simulink model "model_base_bros"  (R2017b)
settings: Solver=FixedStepDiscrete  StartTime=0.0  StopTime=inf  FixedStep=sampleTime  RelTol=1e-3
PostLoadFcn:
  | % load model parameters
  | % pname = fileparts(get_param('model_base_bros','filename'));
  | % run([pname  '\parameters_base_model_bros.m']);
  | parameters_base_model_bros;
  | 
  | % set requested state
  | set_param('model_base_bros/Requested state','Value',num2str(0));
InitFcn:
  | % load model parameters
  | % pname = fileparts(get_param('model_base_bros','filename'));
  | % run([pname  '\parameters_base_model_bros.m']);
  | parameters_base_model_bros;
  | 
  | % set requested state
  | set_param('model_base_bros/Requested state','Value',num2str(0));
StartFcn:
  | % load model parameters
  | % pname = fileparts(get_param('model_base_bros','filename'));
  | % run([pname  '\parameters_base_model_bros.m']);
  | parameters_base_model_bros;
  | 
  | % set requested state
  | set_param('model_base_bros/Requested state','Value',num2str(0));
StopFcn:
  | % switch off data logger (to hopefully avoid corrupt files). TwinCAT doesn't properly switch off the logger when shutting down the model
  | % no idea if this'll work.
  | set_param('model_base_bros/Record data (1 = yes, 0 = no)','Value',num2str(0));
values from neighbouring files (symbols this model uses):
  FFMatrix = -[0 -15; 15 0]    [parameters_base_model_bros.m]
  Lb = 0.07    [parameters_base_model_bros.m]
  Lf = 0.238    [parameters_base_model_bros.m]
  Lu = 0.153    [parameters_base_model_bros.m]
  msin_data_dist1 = [5 11 19 41 59 71 101 137 179 227 0.0358569687947 0.0275584886584 ... (30 elements, 10x3)]    [forcingfunction_data_id.mat]    (also in forcingfunction_data_id_2d_var6_1.mat = [0 0 0 0 0 0 0 0 0 0 0 0 ... (60 elements, 10x6)]; forcingfunction_data_id_2d_var75_nt11.mat = [0 0 0 0 0 0 0 0 0 0 0 0 ... (60 elements, 10x6)]; forcingfunction_data_id_nt10_var6.mat = [5 11 19 41 59 71 101 137 179 227 0.0248424367031 0.01909308)
  msin_data_dist2 = [7 13 23 43 61 73 103 139 181 229 0.0366642780879 0.0272817537998 ... (30 elements, 10x3)]    [forcingfunction_data_id.mat]    (also in forcingfunction_data_id_2d_var6_1.mat = [0 0 0 0 0 0 0 0 0 0 0 0 ... (60 elements, 10x6)]; forcingfunction_data_id_2d_var75_nt11.mat = [0 0 0 0 0 0 0 0 0 0 0 0 ... (60 elements, 10x6)]; forcingfunction_data_id_nt10_var6.mat = [7 13 23 43 61 73 103 139 181 229 0.0254017569884 0.01890135)
  msin_data_target = [2 9 17 27 37 47 0.0347382902327 0.0275101923829 0.0180185190239 0.0110214159229 0.0075682474126 0.00574660779142 ... (18 elements, 6x3)]    [forcingfunction_data_id.mat]    (also in forcingfunction_data_id_2d_var6_1.mat = [5 11 23 37 51 71 101 137 171 226 0.0252651788023 0.01941798; forcingfunction_data_id_2d_var75_nt11.mat = [5 11 23 37 51 71 101 137 173 227 263 0.0282088788597 ... (6; forcingfunction_data_id_nt10_var6.mat = [2 9 17 29 37 47 67 107 149 211 0.0239780224904 0.0189888450; forcingfunction_id_emg.mat = [3 7 13 19 31 0.0450441024419 0.0275859409824 0.015205627144)
  sampleTime = 0.001    [parameters_base_model_bros.m]
  Tm = 81.92    [forcingfunction_data_id_2d_var6_1.mat]    (also in forcingfunction_data_id_2d_var75_nt11.mat; forcingfunction_data_id_nt10_var6.mat; forcingfunction_id_emg.mat = 24)
undefined symbols (not defined in the file or in its folder): BROS1, BROS2, DiscIntNeverNeededParam
libraries: simulink x28, LibraryFM x14, VariousBlocksLibrary x13, simulink_extras x1
(part 3 of 4)

== system model_base_bros/Robot2/DataToEtherCAT/WorkspacePositionGuard ==
  note: Check internal angles
  note: Check whether endpoint position is within the predefined workspace
      | (ellipse)
  note: Check for singularity of joint configuration by checking
      | the condition number. When it exceeds a certain value, go to a safe mode
      | For now, this means disabling the actuators.
      | Note that the boundaries set using admittance should prohibit this from happening.
      | However, if sometjhing really goes wrong, this is a safe guard
  BusRobot : Inport
  StateSystem : Inport  Port=2
  AvoidAlgebraicLoop : Memory
  Bus Selector : BusSelector  OutputSignals=xOpSpace.x,xOpSpace.conditioning,qJointSpace.q_all
  CheckInternalAngles : MATLAB Function  TreatAsAtomicUnit=on
  Compare To Constant : simulink/Logic and Bit Operations/Compare To Constant  relop=>  const=4  OutDataTypeStr=boolean
  Compare To Constant1 : simulink/Logic and Bit Operations/Compare To Constant  relop=>=  const=2.75  OutDataTypeStr=boolean
  Data Type Conversion1 : DataTypeConversion  OutDataTypeStr=boolean
  Data Type Conversion2 : DataTypeConversion  Commented=through  OutDataTypeStr=int32
  Data Type Conversion4 : DataTypeConversion  OutDataTypeStr=boolean
  Detect Change : simulink/Logic and Bit Operations/Detect Change  vinit=0  InputProcessing=Inherited  OutDataTypeStr=boolean
  EndpointPositionGuard : MATLAB Function  TreatAsAtomicUnit=on
  LatchRising : LibraryFM/Utilities/LatchRising  ic=0
  Logical Operator : Logic  Operator=OR  AllPortsSameDT=off  OutDataTypeStr=boolean
  Mux : Mux  Inputs=2
  ShowWorkspaceErrorLatched : Display
  WorkspaceLastError : Display
  WorkspaceError : Outport
  WorkspaceErrorLatched : Outport  Port=2
  wires:
  BusRobot/1 -> Bus Selector/1
  Bus Selector/1 -> EndpointPositionGuard/2(xe)  "<x>"
  LatchRising/1 -> Data Type Conversion2/1
  EndpointPositionGuard/1(error) -> Data Type Conversion1/1
  Mux/1 -> AvoidAlgebraicLoop/1, WorkspaceLastError/1
  Detect Change/1 -> LatchRising/Trigger
  AvoidAlgebraicLoop/1 -> WorkspaceError/1, Detect Change/1, LatchRising/1
  Compare To Constant/1 -> EndpointPositionGuard/1(correctState)
  Bus Selector/2 -> Compare To Constant1/1  "<conditioning>"
  StateSystem/1 -> Compare To Constant/1
  Data Type Conversion2/1 -> WorkspaceErrorLatched/1, ShowWorkspaceErrorLatched/1
  CheckInternalAngles/1(angleError) -> Data Type Conversion4/1
  Bus Selector/3 -> CheckInternalAngles/1(theta)  "<q_all>"
  Data Type Conversion4/1 -> Mux/2
  Logical Operator/1 -> Mux/1
  Data Type Conversion1/1 -> Logical Operator/1
  Compare To Constant1/1 -> Logical Operator/2

== system model_base_bros/Experiment & Haptics/Admittance // Virtual model1/Virtual Model/HoldFirstSampleOnEnable ==
  note: These blocks hold the first sample of the input
      | when the block is enabled (through the action port)
  x : Inport
  Enable : EnablePort  StatesWhenEnabling=reset
  Counter Free-Running : simulink/Sources/Counter Free-Running  NumBits=32  tsamp=-1
  Display : Display
  Memory1 : Memory
  Switch : Switch  Threshold=1
  x0 : Outport
  wires:
  Switch/1 -> Display/1, Memory1/1, x0/1
  Memory1/1 -> Switch/1
  Counter Free-Running/1 -> Switch/2
  x/1 -> Switch/3

== system model_base_bros/Experiment & Haptics/Admittance // Virtual model1/Virtual Model/HoldFirstSampleOnEnable1 ==
  note: These blocks hold the first sample of the input
      | when the block is enabled (through the action port)
  x : Inport
  Enable : EnablePort  StatesWhenEnabling=reset
  Counter Free-Running : simulink/Sources/Counter Free-Running  NumBits=32  tsamp=-1
  Display : Display
  Memory1 : Memory
  Switch : Switch  Threshold=1
  x0 : Outport
  wires:
  Switch/1 -> Display/1, Memory1/1, x0/1
  Memory1/1 -> Switch/1
  Counter Free-Running/1 -> Switch/2
  x/1 -> Switch/3

== system model_base_bros/Robot1/Controller_PD/at home/HoldFirstSampleOnEnable ==
  note: These blocks hold the first sample of the input
      | when the block is enabled (through the action port)
  x : Inport
  Enable : EnablePort  StatesWhenEnabling=reset
  Counter Free-Running : simulink/Sources/Counter Free-Running  NumBits=32  tsamp=-1
  Memory1 : Memory
  Signal Conversion : SignalConversion  OverrideOpt=off
  Switch : Switch  Threshold=1
  x0 : Outport
  wires:
  x/1 -> Switch/3
  Counter Free-Running/1 -> Switch/2
  Memory1/1 -> Switch/1
  Switch/1 -> Signal Conversion/1, Memory1/1
  Signal Conversion/1 -> x0/1

== system model_base_bros/Robot1/DataFromEtherCAT/Calculate Arrange Joint and Op Space/forward kinematics ==
  JointPosition_rad : Inport  PortDimensions=[2 1]
  JointVelocity_rads : Inport  Port=2  PortDimensions=[2 1]
  JointAcceleration_rads2 : Inport  Port=3  PortDimensions=[2 1]
  Je : MATLAB Function  TreatAsAtomicUnit=on
  Jedot : MATLAB Function  TreatAsAtomicUnit=on
  Product : Product  Multiplication=Matrix(*)
  calculate xddot : MATLAB Function  TreatAsAtomicUnit=on
  forward kinematics : MATLAB Function  TreatAsAtomicUnit=on
  x : Outport
  xdot : Outport  Port=2
  xddot : Outport  Port=3
  J : Outport  Port=4
  Jdot : Outport  Port=5
  wires:
  JointPosition_rad/1 -> forward kinematics/1(q), Jedot/1(q), Je/1(q)
  Je/1(Je) -> calculate xddot/3(J), Product/1, J/1
  JointVelocity_rads/1 -> calculate xddot/2(qdot), Product/2, Jedot/2(qdot)
  Jedot/1(Jedot) -> calculate xddot/4(Jdot), Jdot/1
  Product/1 -> xdot/1
  forward kinematics/1(x) -> x/1
  calculate xddot/1(xddot) -> xddot/1
  JointAcceleration_rads2/1 -> calculate xddot/1(qddot)

== system model_base_bros/Robot1/DataFromEtherCAT/Calculate Arrange Joint and Op Space/forward kinematics1 ==
  JointPosition_rad : Inport  PortDimensions=[2 1]
  JointVelocity_rads : Inport  Port=2  PortDimensions=[2 1]
  JointAcceleration_rads2 : Inport  Port=3  PortDimensions=[2 1]
  Je : MATLAB Function  TreatAsAtomicUnit=on
  Jedot : MATLAB Function  TreatAsAtomicUnit=on
  Product : Product  Multiplication=Matrix(*)
  calculate xddot : MATLAB Function  TreatAsAtomicUnit=on
  forward kinematics : MATLAB Function  TreatAsAtomicUnit=on
  x : Outport
  xdot : Outport  Port=2
  xddot : Outport  Port=3
  J : Outport  Port=4
  Jdot : Outport  Port=5
  wires:
  JointPosition_rad/1 -> forward kinematics/1(q), Jedot/1(q), Je/1(q)
  Je/1(Je) -> calculate xddot/3(J), Product/1, J/1
  JointVelocity_rads/1 -> calculate xddot/2(qdot), Product/2, Jedot/2(qdot)
  Jedot/1(Jedot) -> calculate xddot/4(Jdot), Jdot/1
  Product/1 -> xdot/1
  forward kinematics/1(x) -> x/1
  calculate xddot/1(xddot) -> xddot/1
  JointAcceleration_rads2/1 -> calculate xddot/1(qddot)

== system model_base_bros/Robot1/DataFromEtherCAT/FTSensor_K6D27/spikefilter ==
  in : Inport
  Demux : Demux  Outputs=6
  Mux1 : Mux  Inputs=6
  spike filter oeps : Subsystem
  spike filter oeps1 : Subsystem
  spike filter oeps2 : Subsystem
  spike filter oeps3 : Subsystem
  spike filter oeps4 : Subsystem
  spike filter oeps5 : Subsystem
  out : Outport
  wires:
  spike filter oeps1/1(y) -> Mux1/2
  Mux1/1 -> out/1
  in/1 -> Demux/1
  Demux/3 -> spike filter oeps2/1(u)
  spike filter oeps4/1(y) -> Mux1/5
  spike filter oeps/1(y) -> Mux1/1
  Demux/6 -> spike filter oeps5/1(u)
  spike filter oeps5/1(y) -> Mux1/6
  Demux/1 -> spike filter oeps/1(u)
  Demux/2 -> spike filter oeps1/1(u)
  Demux/4 -> spike filter oeps3/1(u)
  Demux/5 -> spike filter oeps4/1(u)
  spike filter oeps2/1(y) -> Mux1/3
  spike filter oeps3/1(y) -> Mux1/4

== system model_base_bros/Robot2/Controller_PD/at home/HoldFirstSampleOnEnable ==
  note: These blocks hold the first sample of the input
      | when the block is enabled (through the action port)
  x : Inport
  Enable : EnablePort  StatesWhenEnabling=reset
  Counter Free-Running : simulink/Sources/Counter Free-Running  NumBits=32  tsamp=-1
  Memory1 : Memory
  Signal Conversion : SignalConversion  OverrideOpt=off
  Switch : Switch  Threshold=1
  x0 : Outport
  wires:
  x/1 -> Switch/3
  Counter Free-Running/1 -> Switch/2
  Memory1/1 -> Switch/1
  Switch/1 -> Signal Conversion/1, Memory1/1
  Signal Conversion/1 -> x0/1

== system model_base_bros/Robot2/DataFromEtherCAT/Calculate Arrange Joint and Op Space/forward kinematics ==
  JointPosition_rad : Inport  PortDimensions=[2 1]
  JointVelocity_rads : Inport  Port=2  PortDimensions=[2 1]
  JointAcceleration_rads2 : Inport  Port=3  PortDimensions=[2 1]
  Je : MATLAB Function  TreatAsAtomicUnit=on
  Jedot : MATLAB Function  TreatAsAtomicUnit=on
  Product : Product  Multiplication=Matrix(*)
  calculate xddot : MATLAB Function  TreatAsAtomicUnit=on
  forward kinematics : MATLAB Function  TreatAsAtomicUnit=on
  x : Outport
  xdot : Outport  Port=2
  xddot : Outport  Port=3
  J : Outport  Port=4
  Jdot : Outport  Port=5
  wires:
  JointPosition_rad/1 -> forward kinematics/1(q), Jedot/1(q), Je/1(q)
  Je/1(Je) -> calculate xddot/3(J), Product/1, J/1
  JointVelocity_rads/1 -> calculate xddot/2(qdot), Product/2, Jedot/2(qdot)
  Jedot/1(Jedot) -> calculate xddot/4(Jdot), Jdot/1
  Product/1 -> xdot/1
  forward kinematics/1(x) -> x/1
  calculate xddot/1(xddot) -> xddot/1
  JointAcceleration_rads2/1 -> calculate xddot/1(qddot)

== system model_base_bros/Robot2/DataFromEtherCAT/Calculate Arrange Joint and Op Space/forward kinematics1 ==
  JointPosition_rad : Inport  PortDimensions=[2 1]
  JointVelocity_rads : Inport  Port=2  PortDimensions=[2 1]
  JointAcceleration_rads2 : Inport  Port=3  PortDimensions=[2 1]
  Je : MATLAB Function  TreatAsAtomicUnit=on
  Jedot : MATLAB Function  TreatAsAtomicUnit=on
  Product : Product  Multiplication=Matrix(*)
  calculate xddot : MATLAB Function  TreatAsAtomicUnit=on
  forward kinematics : MATLAB Function  TreatAsAtomicUnit=on
  x : Outport
  xdot : Outport  Port=2
  xddot : Outport  Port=3
  J : Outport  Port=4
  Jdot : Outport  Port=5
  wires:
  JointPosition_rad/1 -> forward kinematics/1(q), Jedot/1(q), Je/1(q)
  Je/1(Je) -> calculate xddot/3(J), Product/1, J/1
  JointVelocity_rads/1 -> calculate xddot/2(qdot), Product/2, Jedot/2(qdot)
  Jedot/1(Jedot) -> calculate xddot/4(Jdot), Jdot/1
  Product/1 -> xdot/1
  forward kinematics/1(x) -> x/1
  calculate xddot/1(xddot) -> xddot/1
  JointAcceleration_rads2/1 -> calculate xddot/1(qddot)

== system model_base_bros/Robot2/DataFromEtherCAT/FTSensor_K6D27/spikefilter ==
  in : Inport
  Demux : Demux  Outputs=6
  Mux1 : Mux  Inputs=6
  spike filter oeps : Subsystem
  spike filter oeps1 : Subsystem
  spike filter oeps2 : Subsystem
  spike filter oeps3 : Subsystem
  spike filter oeps4 : Subsystem
  spike filter oeps5 : Subsystem
  out : Outport
  wires:
  spike filter oeps1/1(y) -> Mux1/2
  Mux1/1 -> out/1
  in/1 -> Demux/1
  Demux/3 -> spike filter oeps2/1(u)
  spike filter oeps4/1(y) -> Mux1/5
  spike filter oeps/1(y) -> Mux1/1
  Demux/6 -> spike filter oeps5/1(u)
  spike filter oeps5/1(y) -> Mux1/6
  Demux/1 -> spike filter oeps/1(u)
  Demux/2 -> spike filter oeps1/1(u)
  Demux/4 -> spike filter oeps3/1(u)
  Demux/5 -> spike filter oeps4/1(u)
  spike filter oeps2/1(y) -> Mux1/3
  spike filter oeps3/1(y) -> Mux1/4

== system model_base_bros/Robot1/DataFromEtherCAT/FTSensor_K6D27/spikefilter/spike filter oeps ==
  u : Inport
  'oeps' filter : MATLAB Function  TreatAsAtomicUnit=on
  Memory : Memory
  Terminator : Terminator
  diff threshold spike : Constant  Value=FTSensorStruct.ThresholdDiffForceSensorSpike
  y : Outport
  wires:
  'oeps' filter/2(y) -> y/1, Memory/1
  diff threshold spike/1 -> 'oeps' filter/2(diffthr)
  Memory/1 -> 'oeps' filter/3(u_prev)
  u/1 -> 'oeps' filter/1(u)
  'oeps' filter/1(isSpike) -> Terminator/1

== system model_base_bros/Robot1/DataFromEtherCAT/FTSensor_K6D27/spikefilter/spike filter oeps1 ==
  u : Inport
  'oeps' filter : MATLAB Function  TreatAsAtomicUnit=on
  Memory : Memory
  Terminator : Terminator
  diff threshold spike : Constant  Value=FTSensorStruct.ThresholdDiffForceSensorSpike
  y : Outport
  wires:
  'oeps' filter/2(y) -> y/1, Memory/1
  diff threshold spike/1 -> 'oeps' filter/2(diffthr)
  Memory/1 -> 'oeps' filter/3(u_prev)
  u/1 -> 'oeps' filter/1(u)
  'oeps' filter/1(isSpike) -> Terminator/1

== system model_base_bros/Robot1/DataFromEtherCAT/FTSensor_K6D27/spikefilter/spike filter oeps2 ==
  u : Inport
  'oeps' filter : MATLAB Function  TreatAsAtomicUnit=on
  Memory : Memory
  Terminator : Terminator
  diff threshold spike : Constant  Value=FTSensorStruct.ThresholdDiffForceSensorSpike
  y : Outport
  wires:
  'oeps' filter/2(y) -> y/1, Memory/1
  diff threshold spike/1 -> 'oeps' filter/2(diffthr)
  Memory/1 -> 'oeps' filter/3(u_prev)
  u/1 -> 'oeps' filter/1(u)
  'oeps' filter/1(isSpike) -> Terminator/1

== system model_base_bros/Robot1/DataFromEtherCAT/FTSensor_K6D27/spikefilter/spike filter oeps3 ==
  u : Inport
  'oeps' filter : MATLAB Function  TreatAsAtomicUnit=on
  Memory : Memory
  Terminator : Terminator
  diff threshold spike : Constant  Value=FTSensorStruct.ThresholdDiffForceSensorSpike
  y : Outport
  wires:
  'oeps' filter/2(y) -> y/1, Memory/1
  diff threshold spike/1 -> 'oeps' filter/2(diffthr)
  Memory/1 -> 'oeps' filter/3(u_prev)
  u/1 -> 'oeps' filter/1(u)
  'oeps' filter/1(isSpike) -> Terminator/1

== system model_base_bros/Robot1/DataFromEtherCAT/FTSensor_K6D27/spikefilter/spike filter oeps4 ==
  u : Inport
  'oeps' filter : MATLAB Function  TreatAsAtomicUnit=on
  Memory : Memory
  Terminator : Terminator
  diff threshold spike : Constant  Value=FTSensorStruct.ThresholdDiffForceSensorSpike
  y : Outport
  wires:
  'oeps' filter/2(y) -> y/1, Memory/1
  diff threshold spike/1 -> 'oeps' filter/2(diffthr)
  Memory/1 -> 'oeps' filter/3(u_prev)
  u/1 -> 'oeps' filter/1(u)
  'oeps' filter/1(isSpike) -> Terminator/1

== system model_base_bros/Robot1/DataFromEtherCAT/FTSensor_K6D27/spikefilter/spike filter oeps5 ==
  u : Inport
  'oeps' filter : MATLAB Function  TreatAsAtomicUnit=on
  Memory : Memory
  Terminator : Terminator
  diff threshold spike : Constant  Value=FTSensorStruct.ThresholdDiffForceSensorSpike
  y : Outport
  wires:
  'oeps' filter/2(y) -> y/1, Memory/1
  diff threshold spike/1 -> 'oeps' filter/2(diffthr)
  Memory/1 -> 'oeps' filter/3(u_prev)
  u/1 -> 'oeps' filter/1(u)
  'oeps' filter/1(isSpike) -> Terminator/1

== system model_base_bros/Robot2/DataFromEtherCAT/FTSensor_K6D27/spikefilter/spike filter oeps ==
  u : Inport
  'oeps' filter : MATLAB Function  TreatAsAtomicUnit=on
  Memory : Memory
  Terminator : Terminator
  diff threshold spike : Constant  Value=FTSensorStruct.ThresholdDiffForceSensorSpike
  y : Outport
  wires:
  'oeps' filter/2(y) -> y/1, Memory/1
  diff threshold spike/1 -> 'oeps' filter/2(diffthr)
  Memory/1 -> 'oeps' filter/3(u_prev)
  u/1 -> 'oeps' filter/1(u)
  'oeps' filter/1(isSpike) -> Terminator/1

== system model_base_bros/Robot2/DataFromEtherCAT/FTSensor_K6D27/spikefilter/spike filter oeps1 ==
  u : Inport
  'oeps' filter : MATLAB Function  TreatAsAtomicUnit=on
  Memory : Memory
  Terminator : Terminator
  diff threshold spike : Constant  Value=FTSensorStruct.ThresholdDiffForceSensorSpike
  y : Outport
  wires:
  'oeps' filter/2(y) -> y/1, Memory/1
  diff threshold spike/1 -> 'oeps' filter/2(diffthr)
  Memory/1 -> 'oeps' filter/3(u_prev)
  u/1 -> 'oeps' filter/1(u)
  'oeps' filter/1(isSpike) -> Terminator/1

== system model_base_bros/Robot2/DataFromEtherCAT/FTSensor_K6D27/spikefilter/spike filter oeps2 ==
  u : Inport
  'oeps' filter : MATLAB Function  TreatAsAtomicUnit=on
  Memory : Memory
  Terminator : Terminator
  diff threshold spike : Constant  Value=FTSensorStruct.ThresholdDiffForceSensorSpike
  y : Outport
  wires:
  'oeps' filter/2(y) -> y/1, Memory/1
  diff threshold spike/1 -> 'oeps' filter/2(diffthr)
  Memory/1 -> 'oeps' filter/3(u_prev)
  u/1 -> 'oeps' filter/1(u)
  'oeps' filter/1(isSpike) -> Terminator/1

== system model_base_bros/Robot2/DataFromEtherCAT/FTSensor_K6D27/spikefilter/spike filter oeps3 ==
  u : Inport
  'oeps' filter : MATLAB Function  TreatAsAtomicUnit=on
  Memory : Memory
  Terminator : Terminator
  diff threshold spike : Constant  Value=FTSensorStruct.ThresholdDiffForceSensorSpike
  y : Outport
  wires:
  'oeps' filter/2(y) -> y/1, Memory/1
  diff threshold spike/1 -> 'oeps' filter/2(diffthr)
  Memory/1 -> 'oeps' filter/3(u_prev)
  u/1 -> 'oeps' filter/1(u)
  'oeps' filter/1(isSpike) -> Terminator/1

== system model_base_bros/Robot2/DataFromEtherCAT/FTSensor_K6D27/spikefilter/spike filter oeps4 ==
  u : Inport
  'oeps' filter : MATLAB Function  TreatAsAtomicUnit=on
  Memory : Memory
  Terminator : Terminator
  diff threshold spike : Constant  Value=FTSensorStruct.ThresholdDiffForceSensorSpike
  y : Outport
  wires:
  'oeps' filter/2(y) -> y/1, Memory/1
  diff threshold spike/1 -> 'oeps' filter/2(diffthr)
  Memory/1 -> 'oeps' filter/3(u_prev)
  u/1 -> 'oeps' filter/1(u)
  'oeps' filter/1(isSpike) -> Terminator/1

== system model_base_bros/Robot2/DataFromEtherCAT/FTSensor_K6D27/spikefilter/spike filter oeps5 ==
  u : Inport
  'oeps' filter : MATLAB Function  TreatAsAtomicUnit=on
  Memory : Memory
  Terminator : Terminator
  diff threshold spike : Constant  Value=FTSensorStruct.ThresholdDiffForceSensorSpike
  y : Outport
  wires:
  'oeps' filter/2(y) -> y/1, Memory/1
  diff threshold spike/1 -> 'oeps' filter/2(diffthr)
  Memory/1 -> 'oeps' filter/3(u_prev)
  u/1 -> 'oeps' filter/1(u)
  'oeps' filter/1(isSpike) -> Terminator/1

== matlab function model_base_bros/Robot2/Controller_PD/PD + nonlin (op space)/invJ1 ==
  data: x input; J input; y output
function y = invJ(x,J)

y = J.'*x;

== matlab function model_base_bros/Experiment & Haptics/CalculateTrialPerformanceMSE/Calc_RMSE_BROS1 ==
  data: error input; RMSE output
function RMSE = RMSE(error)
% calculate the mean-squared error

persistent N; % number of samples, counter
persistent SSE; % sum of squared of error
if isempty(N), N = 0; end
if isempty(SSE), SSE = 0; end

N = N+1; % new datapoint, increase sample counter

SSE = SSE + norm(error)^2;
RMSE = sqrt(SSE / N);

== matlab function model_base_bros/Robot1/DataFromEtherCAT/Calculate Arrange Joint and Op Space/Condition number ==
  data: J input; C output
function C = conditioning(J)
%#codegen

C = norm(J)*norm(pinv(J));

== matlab function model_base_bros/Robot2/Controller_PD/PD + nonlin (op space)/nonlinear compensation ==
  data: J input; Jdot input; qdot input; tau output; RobotStruct parameter
function tau = n(J,Jdot,qdot,RobotStruct)
% mass matrix
phat = RobotStruct.DynModParams;

% select parameters
me = phat(3);
Fs1 = phat(4);
Fv1 = phat(5);
Fs2 = phat(6);
Fv2 = phat(7);

% % jacobians
% J = func_eq_Je(q(1),q(2),Lf,Lu,Lb);
% Jdot = func_eq_Jedot(q(1),q(2),qdot(1),qdot(2),Lf,Lu,Lb);

% calculate joint space mass matrix;
p = [me;Fs1;Fv1;Fs2;Fv2];

% psi 
Psi = [(J'*Jdot)*qdot [ssign(qdot(1)) qdot(1); 0 0] [0 0; ssign(qdot(2)) qdot(2)]];

% torque
tau = Psi*p;

function x = ssign(u,b)
%% x = ssign(u,b)
% soft sign
if nargin < 2
    b = 8;
end

x = 2./(1+exp(-b*u))-1;

== matlab function model_base_bros/Robot1/DataFromEtherCAT/Calculate Arrange Joint and Op Space/forward kinematics1/Je ==
  data: q input; Je output size=[2 2]; Lf parameter; Lu parameter; Lb parameter
function Je = Je( q, Lf, Lu, Lb)
%#codegen

% Calculate the Jacobian for this particular device configuration.
% Note that the function func_eq_Je needs to be in the libraries/kinematis_functions folder

% jacobians
Je = func_eq_Je(q(1),q(2),Lf,Lu,Lb);

== matlab function model_base_bros/Robot1/DataFromEtherCAT/Calculate Arrange Joint and Op Space/forward kinematics1/Jedot ==
  data: q input; qdot input; Jedot output size=[2 2]; Lf parameter; Lu parameter; Lb parameter
function Jedot = Jedot( q, qdot, Lf, Lu, Lb)
%#codegen

% Calculate the time derivative of the Jacobian for this particular device configuration.
% Note that the function func_eq_Je needs to be in the libraries/kinematis_functions folder


% jacobians
Jedot = func_eq_Jedot(q(1),q(2),qdot(1),qdot(2),Lf,Lu,Lb);

== matlab function model_base_bros/Robot1/DataFromEtherCAT/Calculate Arrange Joint and Op Space/forward kinematics1/calculate xddot ==
  data: qddot input; qdot input size=[2 1]; J input; xddot output size=[2 1]; Jdot input
function xddot = calc_xddot(qddot, qdot, J, Jdot)
%#codegen

xddot = J*qddot + Jdot*qdot;

== matlab function model_base_bros/Robot2/DataFromEtherCAT/Calculate Arrange Joint and Op Space/Condition number ==
  data: J input; C output
function C = conditioning(J)
%#codegen

C = norm(J)*norm(pinv(J));

== matlab function model_base_bros/Experiment & Haptics/ msin_target ==
  data: time input; T input; time_rand input; msin_data input; p output; v output; a output; Tm input
function [p, v, a]  = msin (time, T, time_rand, msin_data,Tm) 

nx = msin_data(:,1);
Ax = msin_data(:,2);
phx = msin_data(:,3);
ny = msin_data(:,4);
Ay = msin_data(:,5);
phy = msin_data(:,6);

% prepare frequencies
dw = 2*pi/Tm; %w0 depends on trial duration
wx = dw*nx;
wy = dw*ny;

% calculate position, velocity, acceleration
p = [0;0];
v = [0;0];
a = [0;0];

% randomization
% for every multiple of 20, rotate the target signal
% nRand = floor(time_rand/T);
% if nRand > 5, nRand = 5; end

% % add random starting time (semi-randomization)
time = time + mod(time_rand,T);

% calculate sum-of-sines
for i = 1:length(wx)
    % position
    p(1) = p(1) + Ax(i)*sin(wx(i)*time+phx(i));
    p(2) = p(2) + Ay(i)*sin(wy(i)*time+phy(i));
    
    % velocity
    v(1) = v(1) + Ax(i)*wx(i)*cos(wx(i)*time+phx(i));
    v(2) = v(2) + Ay(i)*wy(i)*cos(wy(i)*time+phy(i));
    
    % acceleration
    a(1) = a(1) - Ax(i)*wx(i)^2*sin(wx(i)*time+phx(i));
    a(2) = a(2) - Ay(i)*wy(i)^2*sin(wy(i)*time+phy(i));
end

% due to the difference in coordiante systems (of human reaching, y
% forward, x to the right; robot: y towards you and x to the left), rotate
% the target such that it is in a human-centered coordinate system.
p = -p;
v = -v;
a = -a;

% % rotate target (to make it more random-appearing)
% thetaRot = nRand*(2*pi/6);
% 
% R = [cos(thetaRot) -sin(thetaRot); sin(thetaRot) cos(thetaRot)];
% 
% p = R*p;
% v = R*v;
% a = R*a;

end

== matlab function model_base_bros/Robot1/DataFromEtherCAT/Calculate Arrange Joint and Op Space/forward kinematics/forward kinematics ==
  data: q input; x output size=[2 1]; Lf parameter; Lu parameter; Lb parameter
function x = FK(q, Lf, Lu, Lb)
%#codegen

% Calculate the endpoint position (forward kinematics)
% Note that the function func_eq_FK needs to be in the libraries/kinematis_functions folder


x = func_eq_FK(q(1),q(2),Lf,Lu,Lb);

== matlab function model_base_bros/Robot1/DataFromEtherCAT/Calculate Arrange Joint and Op Space/forward kinematics1/forward kinematics ==
  data: q input; x output size=[2 1]; Lf parameter; Lu parameter; Lb parameter
function x = FK(q, Lf, Lu, Lb)
%#codegen

% Calculate the endpoint position (forward kinematics)
% Note that the function func_eq_FK needs to be in the libraries/kinematis_functions folder


x = func_eq_FK(q(1),q(2),Lf,Lu,Lb);

== matlab function model_base_bros/Robot1/DataToEtherCAT/FTSensorError/MATLAB Function ==
  data: ForcesTorques input; e output; MaxForcesTorques input
function e = fcn(ForcesTorques, MaxForcesTorques)

% throw error when any of the forces/torques go over a max allowable value
if any(abs(ForcesTorques) > MaxForcesTorques) 
    e = 1;
else
    e = 0;
end

== matlab function model_base_bros/Robot1/Controller_PD/PD + nonlin (op space)/invJ1 ==
  data: x input; J input; y output
function y = invJ(x,J)

y = J.'*x;

== matlab function model_base_bros/Robot2/DataFromEtherCAT/Calculate Arrange Joint and Op Space/IK all joints ==
  data: x input; q_all output; Lf parameter; Lu parameter; Lb parameter
function q_all = IK_all(x,Lf,Lu,Lb)
%#codegen

q_all = func_eqs_IK_all(x(1),x(2),Lf,Lu,Lb);

if any(isnan(q_all)) || any(isinf(q_all))
    q_all = zeros(5,1);
end

== matlab function model_base_bros/Robot2/DataFromEtherCAT/Calculate Arrange Joint and Op Space/forward kinematics/Je ==
  data: q input; Je output size=[2 2]; Lf parameter; Lu parameter; Lb parameter
function Je = Je( q, Lf, Lu, Lb)
%#codegen

% Calculate the Jacobian for this particular device configuration.
% Note that the function func_eq_Je needs to be in the libraries/kinematis_functions folder

% jacobians
Je = func_eq_Je(q(1),q(2),Lf,Lu,Lb);

== matlab function model_base_bros/Robot2/DataFromEtherCAT/Calculate Arrange Joint and Op Space/forward kinematics/Jedot ==
  data: q input; qdot input; Jedot output size=[2 2]; Lf parameter; Lu parameter; Lb parameter
function Jedot = Jedot( q, qdot, Lf, Lu, Lb)
%#codegen

% Calculate the time derivative of the Jacobian for this particular device configuration.
% Note that the function func_eq_Je needs to be in the libraries/kinematis_functions folder


% jacobians
Jedot = func_eq_Jedot(q(1),q(2),qdot(1),qdot(2),Lf,Lu,Lb);

== matlab function model_base_bros/Robot2/DataFromEtherCAT/Calculate Arrange Joint and Op Space/forward kinematics/calculate xddot ==
  data: qddot input; qdot input size=[2 1]; J input; xddot output size=[2 1]; Jdot input
function xddot = calc_xddot(qddot, qdot, J, Jdot)
%#codegen

xddot = J*qddot + Jdot*qdot;

== matlab function model_base_bros/Robot2/DataFromEtherCAT/Calculate Arrange Joint and Op Space/forward kinematics/forward kinematics ==
  data: q input; x output size=[2 1]; Lf parameter; Lu parameter; Lb parameter
function x = FK(q, Lf, Lu, Lb)
%#codegen

% Calculate the endpoint position (forward kinematics)
% Note that the function func_eq_FK needs to be in the libraries/kinematis_functions folder


x = func_eq_FK(q(1),q(2),Lf,Lu,Lb);

== matlab function model_base_bros/Robot1/DataFromEtherCAT/Calculate Arrange Joint and Op Space/forward kinematics/Je ==
  data: q input; Je output size=[2 2]; Lf parameter; Lu parameter; Lb parameter
function Je = Je( q, Lf, Lu, Lb)
%#codegen

% Calculate the Jacobian for this particular device configuration.
% Note that the function func_eq_Je needs to be in the libraries/kinematis_functions folder

% jacobians
Je = func_eq_Je(q(1),q(2),Lf,Lu,Lb);

== matlab function model_base_bros/Robot1/DataFromEtherCAT/Calculate Arrange Joint and Op Space/forward kinematics/Jedot ==
  data: q input; qdot input; Jedot output size=[2 2]; Lf parameter; Lu parameter; Lb parameter
function Jedot = Jedot( q, qdot, Lf, Lu, Lb)
%#codegen

% Calculate the time derivative of the Jacobian for this particular device configuration.
% Note that the function func_eq_Je needs to be in the libraries/kinematis_functions folder


% jacobians
Jedot = func_eq_Jedot(q(1),q(2),qdot(1),qdot(2),Lf,Lu,Lb);

== matlab function model_base_bros/Robot1/DataFromEtherCAT/FTSensor_K6D27/CorrectOffset ==
  data: u_in input; u_out output; reset input; corrected output
function [u_out,corrected] = CorrectOffset(u_in,reset)
%#codegen

persistent data_ offset_ counter_ corrected_;
N = 1000;

% initialize
if isempty(data_)
    data_ = zeros(size(u_in,1), N);
    offset_ = zeros(size(u_in));
    counter_ = 1;
    corrected_ = 0;
end

if (counter_ <= N)
    data_(:,counter_) = u_in;
end

counter_ = counter_ + 1;
if reset
    counter_ = 1;
end

% calculate mean
if counter_ == N
    corrected_ = 1;
    offset_ = mean(data_,2);
end

corrected = corrected_;
u_out = u_in - offset_;

== matlab function model_base_bros/Robot2/DataFromEtherCAT/Calculate Arrange Joint and Op Space/forward kinematics1/Je ==
  data: q input; Je output size=[2 2]; Lf parameter; Lu parameter; Lb parameter
function Je = Je( q, Lf, Lu, Lb)
%#codegen

% Calculate the Jacobian for this particular device configuration.
% Note that the function func_eq_Je needs to be in the libraries/kinematis_functions folder

% jacobians
Je = func_eq_Je(q(1),q(2),Lf,Lu,Lb);

== matlab function model_base_bros/Robot1/DataFromEtherCAT/Calculate Arrange Joint and Op Space/IK all joints ==
  data: x input; q_all output; Lf parameter; Lu parameter; Lb parameter
function q_all = IK_all(x,Lf,Lu,Lb)
%#codegen

q_all = func_eqs_IK_all(x(1),x(2),Lf,Lu,Lb);

if any(isnan(q_all)) || any(isinf(q_all))
    q_all = zeros(5,1);
end

== matlab function model_base_bros/Robot1/DataFromEtherCAT/Calculate Arrange Joint and Op Space/forward kinematics/calculate xddot ==
  data: qddot input; qdot input size=[2 1]; J input; xddot output size=[2 1]; Jdot input
function xddot = calc_xddot(qddot, qdot, J, Jdot)
%#codegen

xddot = J*qddot + Jdot*qdot;

== matlab function model_base_bros/Robot2/DataFromEtherCAT/Calculate Arrange Joint and Op Space/forward kinematics1/Jedot ==
  data: q input; qdot input; Jedot output size=[2 2]; Lf parameter; Lu parameter; Lb parameter
function Jedot = Jedot( q, qdot, Lf, Lu, Lb)
%#codegen

% Calculate the time derivative of the Jacobian for this particular device configuration.
% Note that the function func_eq_Je needs to be in the libraries/kinematis_functions folder


% jacobians
Jedot = func_eq_Jedot(q(1),q(2),qdot(1),qdot(2),Lf,Lu,Lb);

== matlab function model_base_bros/Robot1/Controller_PD/PD + nonlin (op space)/nonlinear compensation ==
  data: J input; Jdot input; qdot input; tau output; RobotStruct parameter
function tau = n(J,Jdot,qdot,RobotStruct)
% mass matrix
phat = RobotStruct.DynModParams;

% select parameters
me = phat(3);
Fs1 = phat(4);
Fv1 = phat(5);
Fs2 = phat(6);
Fv2 = phat(7);

% % jacobians
% J = func_eq_Je(q(1),q(2),Lf,Lu,Lb);
% Jdot = func_eq_Jedot(q(1),q(2),qdot(1),qdot(2),Lf,Lu,Lb);

% calculate joint space mass matrix;
p = [me;Fs1;Fv1;Fs2;Fv2];

% psi 
Psi = [(J'*Jdot)*qdot [ssign(qdot(1)) qdot(1); 0 0] [0 0; ssign(qdot(2)) qdot(2)]];

% torque
tau = Psi*p;

function x = ssign(u,b)
%% x = ssign(u,b)
% soft sign
if nargin < 2
    b = 8;
end

x = 2./(1+exp(-b*u))-1;

== matlab function model_base_bros/Robot2/DataFromEtherCAT/Calculate Arrange Joint and Op Space/forward kinematics1/calculate xddot ==
  data: qddot input; qdot input size=[2 1]; J input; xddot output size=[2 1]; Jdot input
function xddot = calc_xddot(qddot, qdot, J, Jdot)
%#codegen

xddot = J*qddot + Jdot*qdot;

== matlab function model_base_bros/Robot2/DataFromEtherCAT/Calculate Arrange Joint and Op Space/forward kinematics1/forward kinematics ==
  data: q input; x output size=[2 1]; Lf parameter; Lu parameter; Lb parameter
function x = FK(q, Lf, Lu, Lb)
%#codegen

% Calculate the endpoint position (forward kinematics)
% Note that the function func_eq_FK needs to be in the libraries/kinematis_functions folder


x = func_eq_FK(q(1),q(2),Lf,Lu,Lb);

== matlab function model_base_bros/Robot2/DataFromEtherCAT/FTSensor_K6D27/CorrectOffset ==
  data: u_in input; u_out output; reset input; corrected output
function [u_out,corrected] = CorrectOffset(u_in,reset)
%#codegen

persistent data_ offset_ counter_ corrected_;
N = 1000;

% initialize
if isempty(data_)
    data_ = zeros(size(u_in,1), N);
    offset_ = zeros(size(u_in));
    counter_ = 1;
    corrected_ = 0;
end

if (counter_ <= N)
    data_(:,counter_) = u_in;
end

counter_ = counter_ + 1;
if reset
    counter_ = 1;
end

% calculate mean
if counter_ == N
    corrected_ = 1;
    offset_ = mean(data_,2);
end

corrected = corrected_;
u_out = u_in - offset_;

== matlab function model_base_bros/Robot2/DataFromEtherCAT/FTSensor_K6D27/SensorToOperationalSpace ==
  data: q_all input; Fs input; FTOpSpace output; transmatside input
function FTOpSpace = ForceSensorToOperationalSpace(q_all,Fs,transmatside)
%#codegen
q1 = q_all(1);
q2 = q_all(2);
q4 = q_all(4);
q5 = q_all(5);

% based on which arm the force sensor is connected
switch transmatside
    case 1
        alpha = pi-q2;   
        beta = q1+alpha-pi/2;
        R0 = rotmat(beta);
        R = blkdiag(R0,R0); % transform forces and moments
    case 2
        alpha = -(pi - q4);
        beta = q5+alpha-pi/2;
        R0 = rotmat(beta);
        R = blkdiag(R0,R0); % transform forces and moments
    otherwise
        R = eye(length(Fs));
end

% transform force
FTOpSpace = R*Fs;

function R = rotmat(q)

R = [cos(q) -sin(q) 0;...
      sin(q)  cos(q) 0;...
      0       0      1];

== matlab function model_base_bros/Robot2/DataToEtherCAT/CreateSingleErrorValue1/ErrorToPower2 ==
  data: u input; e output
function e = errorToPowerOf2(u)

e = (2.^(0:length(u)-1))*u;

== matlab function model_base_bros/Robot2/DataToEtherCAT/CreateSingleErrorValue2/ErrorToPower2 ==
  data: u input; e output
function e = errorToPowerOf2(u)

e = (2.^(0:length(u)-1))*u;

== matlab function model_base_bros/Robot2/DataToEtherCAT/FTSensorError/MATLAB Function ==
  data: ForcesTorques input; e output; MaxForcesTorques input
function e = fcn(ForcesTorques, MaxForcesTorques)

% throw error when any of the forces/torques go over a max allowable value
if any(abs(ForcesTorques) > MaxForcesTorques) 
    e = 1;
else
    e = 0;
end

== matlab function model_base_bros/Robot2/DataToEtherCAT/WorkspacePositionGuard/CheckInternalAngles ==
  data: theta input; angleError output
function angleError = checkInternalErrors(theta)
%#codegen


angleError = 0;
if any(theta([2 4]) >= 0.95*pi)
    angleError = 1;
end

== matlab function model_base_bros/Robot2/DataToEtherCAT/WorkspacePositionGuard/EndpointPositionGuard ==
  data: correctState input; xe input; error output
function error = fcn(correctState, xe)
%#codegen


error = 0;

% only check workspace boundaries after homing state is done
if ~correctState 
    return; 
end

% x0 = 0;
% y0 = 0.2354;
% a = 0.11;
% b = 0.08;

% workspace (see design document)
x0 = 0;
y0 = 0.25024;
a = 0.1746;
b = 0.13;%0.1048;

% check if endpoint is outside a predefined ellipse
x = xe(1);
y = xe(2);

% workspace is defined as an ellipse
e = (x-x0)^2 / a^2 + (y-y0)^2 / b^2;

% if is larger than 1, the endpoint is outside the workspace
if e > 1
    error = 1;
end

== matlab function model_base_bros/Robot2/DataFromEtherCAT/FTSensor_K6D27/spikefilter/spike filter oeps/'oeps' filter ==
  data: isSpike output; u input; diffthr input; y output; u_prev input
function [isSpike,y] = fcn(u,diffthr,u_prev)
du = u-u_prev;
isSpike = 0;
if (abs(du) > diffthr)
    y = u_prev+sign(du)*diffthr;
    isSpike = 1;
else
    y = u;
end

== matlab function model_base_bros/Robot2/DataFromEtherCAT/FTSensor_K6D27/spikefilter/spike filter oeps1/'oeps' filter ==
  data: isSpike output; u input; diffthr input; y output; u_prev input
function [isSpike,y] = fcn(u,diffthr,u_prev)
du = u-u_prev;
isSpike = 0;
if (abs(du) > diffthr)
    y = u_prev+sign(du)*diffthr;
    isSpike = 1;
else
    y = u;
end

== matlab function model_base_bros/Robot2/DataFromEtherCAT/FTSensor_K6D27/spikefilter/spike filter oeps2/'oeps' filter ==
  data: isSpike output; u input; diffthr input; y output; u_prev input
function [isSpike,y] = fcn(u,diffthr,u_prev)
du = u-u_prev;
isSpike = 0;
if (abs(du) > diffthr)
    y = u_prev+sign(du)*diffthr;
    isSpike = 1;
else
    y = u;
end

== matlab function model_base_bros/Experiment & Haptics/CalculateTrialPerformanceMSE/Calc_RMSE_BROS2 ==
  data: error input; RMSE output
function RMSE = RMSE(error)
% calculate the mean-squared error

persistent N; % number of samples, counter
persistent SSE; % sum of squared of error
if isempty(N), N = 0; end
if isempty(SSE), SSE = 0; end

N = N+1; % new datapoint, increase sample counter

SSE = SSE + norm(error)^2;
RMSE = sqrt(SSE / N);

== matlab function model_base_bros/Robot2/DataFromEtherCAT/FTSensor_K6D27/spikefilter/spike filter oeps3/'oeps' filter ==
  data: isSpike output; u input; diffthr input; y output; u_prev input
function [isSpike,y] = fcn(u,diffthr,u_prev)
du = u-u_prev;
isSpike = 0;
if (abs(du) > diffthr)
    y = u_prev+sign(du)*diffthr;
    isSpike = 1;
else
    y = u;
end

== matlab function model_base_bros/Robot1/DataToEtherCAT/CreateSingleErrorValue2/ErrorToPower2 ==
  data: u input; e output
function e = errorToPowerOf2(u)

e = (2.^(0:length(u)-1))*u;

== matlab function model_base_bros/Robot1/DataToEtherCAT/CreateSingleErrorValue1/ErrorToPower2 ==
  data: u input; e output
function e = errorToPowerOf2(u)

e = (2.^(0:length(u)-1))*u;

== matlab function model_base_bros/Robot2/DataFromEtherCAT/FTSensor_K6D27/spikefilter/spike filter oeps4/'oeps' filter ==
  data: isSpike output; u input; diffthr input; y output; u_prev input
function [isSpike,y] = fcn(u,diffthr,u_prev)
du = u-u_prev;
isSpike = 0;
if (abs(du) > diffthr)
    y = u_prev+sign(du)*diffthr;
    isSpike = 1;
else
    y = u;
end

== matlab function model_base_bros/Robot1/DataFromEtherCAT/FTSensor_K6D27/SensorToOperationalSpace ==
  data: q_all input; Fs input; FTOpSpace output; transmatside input
function FTOpSpace = ForceSensorToOperationalSpace(q_all,Fs,transmatside)
%#codegen
q1 = q_all(1);
q2 = q_all(2);
q4 = q_all(4);
q5 = q_all(5);

% based on which arm the force sensor is connected
switch transmatside
    case 1
        alpha = pi-q2;   
        beta = q1+alpha-pi/2;
        R0 = rotmat(beta);
        R = blkdiag(R0,R0); % transform forces and moments
    case 2
        alpha = -(pi - q4);
        beta = q5+alpha-pi/2;
        R0 = rotmat(beta);
        R = blkdiag(R0,R0); % transform forces and moments
    otherwise
        R = eye(length(Fs));
end

% transform force
FTOpSpace = R*Fs;

function R = rotmat(q)

R = [cos(q) -sin(q) 0;...
      sin(q)  cos(q) 0;...
      0       0      1];

== matlab function model_base_bros/Experiment & Haptics/Admittance // Virtual model1/Virtual Model/Virtual model ==
  data: divTs input; x1 output; xdot1 output; xddot1 output; x2 output size=[2 1]; xdot2 output; xddot2 output; M_v input; B_v input; F1 input; F2 input; x0_1 input; x0_2 input; x1_nompos input; x2_nompos input; Kp_s input; Kd_s input; isConnected input; FFMatrix input; doForceField input; constrainY input; x1_prev input size=2; xdot1_prev input size=2; x2_prev input; xdot2_prev input; sampleTime parameter; Fs1 output; Fs2 output
function [x1,xdot1,xddot1,x2,xdot2,xddot2,Fs1,Fs2] = AC(divTs, M_v, B_v, F1, F2, x0_1, x0_2, x1_nompos,x2_nompos,Kp_s,Kd_s,isConnected,FFMatrix,doForceField,constrainY,x1_prev, xdot1_prev, x2_prev, xdot2_prev, sampleTime)



% constants & limits
div_Ts = max(1,divTs);
Ts = sampleTime/div_Ts;
maxRadius = 0.1;
maxVel = 2.0;
maxAcc = 100.0;
maxForceSpring = 50;
b_b = 0.5; % damping on boundary

% persistents
persistent x1_prev_tmp;
persistent x2_prev_tmp;
persistent onBoundary1;
persistent onBoundary2;

if isempty(x1_prev_tmp), x1_prev_tmp = x0_1;
else, x1_prev_tmp = x1_prev; end 

if isempty(x2_prev_tmp), x2_prev_tmp = x0_2;
else, x2_prev_tmp = x2_prev; end 

if isempty(onBoundary1), onBoundary1 = 0; end
if isempty(onBoundary2), onBoundary2 = 0; end

% lower bounds to mass and damping
m_v = max(0.1,M_v); %lower bound M_v
b_v = max(0,B_v);

if length(m_v) == 1
    m_v1 = m_v;
    m_v2 = m_v;
else
    m_v1 = m_v(1);
    m_v2 = m_v(2);
end

if length(b_v) == 1
    b_v1 = b_v;
    b_v2 = b_v;
else
    b_v1 = b_v(1);
    b_v2 = b_v(2);
end

% assign previous values to x1, x2, xdot1 etc
x1 = x1_prev;
x2 = x2_prev;
xdot1 = xdot1_prev;
xdot2 = xdot1_prev;
xddot1 = [0;0];
xddot2 = [0;0];
Fs1 = [0;0];
Fs2 = [0;0];
% perform integration of virtual dynamics
% using semi-implicit Euler integration

for ii = 1:div_Ts
    % calculate acceleration

    % spring force
    Fs1 = Kp_s*(x2_prev - x1_prev) + Kd_s*(xdot2_prev - xdot1_prev);
    Fs1 = limit(Fs1,maxForceSpring);
    Fs2 = Kp_s*(x1_prev - x2_prev) + Kd_s*(xdot1_prev - xdot2_prev);
    Fs2 = limit(Fs2,maxForceSpring);
    
    if constrainY
        Fs1(2) = 0; 
        Fs2(2) = 0;
    end
    
    % force field
    
    % BROS 1
    xddot1 = (F1 + isConnected*Fs1 + doForceField*FFMatrix*xdot1_prev - b_v1*xdot1_prev - onBoundary1*b_b*xdot1_prev)/m_v1;
    xddot1 = limit(xddot1,maxAcc);

    % BROS 2
    xddot2 = (F2 + isConnected*Fs2 + doForceField*FFMatrix*xdot2_prev - b_v2*xdot2_prev - onBoundary2*b_b*xdot2_prev)/m_v2;
    xddot2 = limit(xddot2,maxAcc);
    
    if constrainY
        xddot1(2) = 0; 
        xddot2(2) = 0;
    end

    % acc -> vel
    % BROS 1
    xdot1 = xdot1_prev + xddot1*Ts;
    [xdot1,lim_vel] = limit(xdot1,maxVel);
    if (lim_vel)
        xddot1 = [0;0];
    end

    % BROS 2
    xdot2 = xdot2_prev + xddot2*Ts;
    [xdot2,lim_vel] = limit(xdot2,maxVel);
    if (lim_vel)
        xddot2 = [0;0];
    end
    
    if constrainY
        xdot1(2) = 0; 
        xdot2(2) = 0;
    end

    % vel -> pos
    % BROS 1
    x1 = x1_prev_tmp + xdot1*Ts;

    [x1,lim_pos] = limit(x1-x1_nompos,maxRadius);
    if (lim_pos)
        onBoundary1 = 1;
        unitVec = x1/norm(x1);
        xdot1 = xdot1 - dot(unitVec,xdot1)*unitVec;     % remove normal component
        xddot1 = xddot1 - dot(unitVec,xddot1)*unitVec;  % remove normal component 
    else
        onBoundary1 = 0;
    end
    x1 = x1 + x1_nompos;

    % BROS 2
    x2 = x2_prev_tmp + xdot2*Ts;

    [x2,lim_pos] = limit(x2-x2_nompos,maxRadius);
    if (lim_pos)
        onBoundary2 = 1;
        unitVec = x2/norm(x2);
        xdot2 = xdot2 - dot(unitVec,xdot2)*unitVec;     % remove normal component
        xddot2 = xddot2 - dot(unitVec,xddot2)*unitVec;  % remove normal component 
    else
        onBoundary2 = 0;
    end
    x2 = x2 + x2_nompos;
    
    x1_prev_tmp = x1;
    x2_prev_tmp = x2;
    xdot1_prev = xdot1;
    xdot2_prev = xdot2;
end

end

% limit
function [y,lim] = limit(x,maxVal)
    vecLen = norm(x);
    if vecLen > maxVal
        y = x / vecLen * maxVal;
        lim = 1; 
    else
        y = x;
        lim = 0;
    end
end

== matlab function model_base_bros/Robot1/DataToEtherCAT/WorkspacePositionGuard/CheckInternalAngles ==
  data: theta input; angleError output
function angleError = checkInternalErrors(theta)
%#codegen


angleError = 0;
if any(theta([2 4]) >= 0.95*pi)
    angleError = 1;
end

== matlab function model_base_bros/Robot2/DataFromEtherCAT/FTSensor_K6D27/spikefilter/spike filter oeps5/'oeps' filter ==
  data: isSpike output; u input; diffthr input; y output; u_prev input
function [isSpike,y] = fcn(u,diffthr,u_prev)
du = u-u_prev;
isSpike = 0;
if (abs(du) > diffthr)
    y = u_prev+sign(du)*diffthr;
    isSpike = 1;
else
    y = u;
end

== matlab function model_base_bros/Robot1/DataToEtherCAT/WorkspacePositionGuard/EndpointPositionGuard ==
  data: correctState input; xe input; error output
function error = fcn(correctState, xe)
%#codegen


error = 0;

% only check workspace boundaries after homing state is done
if ~correctState 
    return; 
end

% x0 = 0;
% y0 = 0.2354;
% a = 0.11;
% b = 0.08;

% workspace (see design document)
x0 = 0;
y0 = 0.25024;
a = 0.1746;
b = 0.13;%0.1048;

% check if endpoint is outside a predefined ellipse
x = xe(1);
y = xe(2);

% workspace is defined as an ellipse
e = (x-x0)^2 / a^2 + (y-y0)^2 / b^2;

% if is larger than 1, the endpoint is outside the workspace
if e > 1
    error = 1;
end

== matlab function model_base_bros/Robot1/DataFromEtherCAT/FTSensor_K6D27/spikefilter/spike filter oeps/'oeps' filter ==
  data: isSpike output; u input; diffthr input; y output; u_prev input
function [isSpike,y] = fcn(u,diffthr,u_prev)
du = u-u_prev;
isSpike = 0;
if (abs(du) > diffthr)
    y = u_prev+sign(du)*diffthr;
    isSpike = 1;
else
    y = u;
end

== matlab function model_base_bros/Robot1/DataFromEtherCAT/FTSensor_K6D27/spikefilter/spike filter oeps1/'oeps' filter ==
  data: isSpike output; u input; diffthr input; y output; u_prev input
function [isSpike,y] = fcn(u,diffthr,u_prev)
du = u-u_prev;
isSpike = 0;
if (abs(du) > diffthr)
    y = u_prev+sign(du)*diffthr;
    isSpike = 1;
else
    y = u;
end

== matlab function model_base_bros/Robot1/DataFromEtherCAT/FTSensor_K6D27/spikefilter/spike filter oeps2/'oeps' filter ==
  data: isSpike output; u input; diffthr input; y output; u_prev input
function [isSpike,y] = fcn(u,diffthr,u_prev)
du = u-u_prev;
isSpike = 0;
if (abs(du) > diffthr)
    y = u_prev+sign(du)*diffthr;
    isSpike = 1;
else
    y = u;
end

== matlab function model_base_bros/Robot1/DataFromEtherCAT/FTSensor_K6D27/spikefilter/spike filter oeps3/'oeps' filter ==
  data: isSpike output; u input; diffthr input; y output; u_prev input
function [isSpike,y] = fcn(u,diffthr,u_prev)
du = u-u_prev;
isSpike = 0;
if (abs(du) > diffthr)
    y = u_prev+sign(du)*diffthr;
    isSpike = 1;
else
    y = u;
end

== matlab function model_base_bros/Robot1/DataFromEtherCAT/FTSensor_K6D27/spikefilter/spike filter oeps4/'oeps' filter ==
  data: isSpike output; u input; diffthr input; y output; u_prev input
function [isSpike,y] = fcn(u,diffthr,u_prev)
du = u-u_prev;
isSpike = 0;
if (abs(du) > diffthr)
    y = u_prev+sign(du)*diffthr;
    isSpike = 1;
else
    y = u;
end

== matlab function model_base_bros/Robot1/DataFromEtherCAT/FTSensor_K6D27/spikefilter/spike filter oeps5/'oeps' filter ==
  data: isSpike output; u input; diffthr input; y output; u_prev input
function [isSpike,y] = fcn(u,diffthr,u_prev)
du = u-u_prev;
isSpike = 0;
if (abs(du) > diffthr)
    y = u_prev+sign(du)*diffthr;
    isSpike = 1;
else
    y = u;
end

== matlab function model_base_bros/Experiment & Haptics/msin_dist1 ==
  data: time input; T input; time_rand input; msin_data input; p output; v output; a output; Tm input
function [p, v, a]  = msin (time, T, time_rand, msin_data,Tm) 

nx = msin_data(:,1);
Ax = msin_data(:,2);
phx = msin_data(:,3);
ny = msin_data(:,4);
Ay = msin_data(:,5);
phy = msin_data(:,6);

% prepare frequencies
dw = 2*pi/Tm; %w0 depends on trial duration
wx = dw*nx;
wy = dw*ny;

% calculate position, velocity, acceleration
p = [0;0];
v = [0;0];
a = [0;0];

% randomization
% for every multiple of 20, rotate the target signal
% nRand = floor(time_rand/T);
% if nRand > 5, nRand = 5; end

% % add random starting time (semi-randomization)
time = time + mod(time_rand,T);

% calculate sum-of-sines
for i = 1:length(wx)
    % position
    p(1) = p(1) + Ax(i)*sin(wx(i)*time+phx(i));
    p(2) = p(2) + Ay(i)*sin(wy(i)*time+phy(i));
    
    % velocity
    v(1) = v(1) + Ax(i)*wx(i)*cos(wx(i)*time+phx(i));
    v(2) = v(2) + Ay(i)*wy(i)*cos(wy(i)*time+phy(i));
    
    % acceleration
    a(1) = a(1) - Ax(i)*wx(i)^2*sin(wx(i)*time+phx(i));
    a(2) = a(2) - Ay(i)*wy(i)^2*sin(wy(i)*time+phy(i));
end

% due to the difference in coordiante systems (of human reaching, y
% forward, x to the right; robot: y towards you and x to the left), rotate
% the target such that it is in a human-centered coordinate system.
p = -p;
v = -v;
a = -a;

% % rotate target (to make it more random-appearing)
% thetaRot = nRand*(2*pi/6);
% 
% R = [cos(thetaRot) -sin(thetaRot); sin(thetaRot) cos(thetaRot)];
% 
% p = R*p;
% v = R*v;
% a = R*a;

end
